simulink model "RGB_Color_Component_ManualThresholding"  (R2016a)
settings: Solver=VariableStepAuto  StartTime=0.0  StopTime=inf  RelTol=1e-3
undefined symbols (not defined in the file): none, Rec, SDTV, videoinput
libraries: visionconversions x2, imaqlib x1, visionsinks x1
settings Model: Creator=YASARA  LastModifiedBy=YASARA

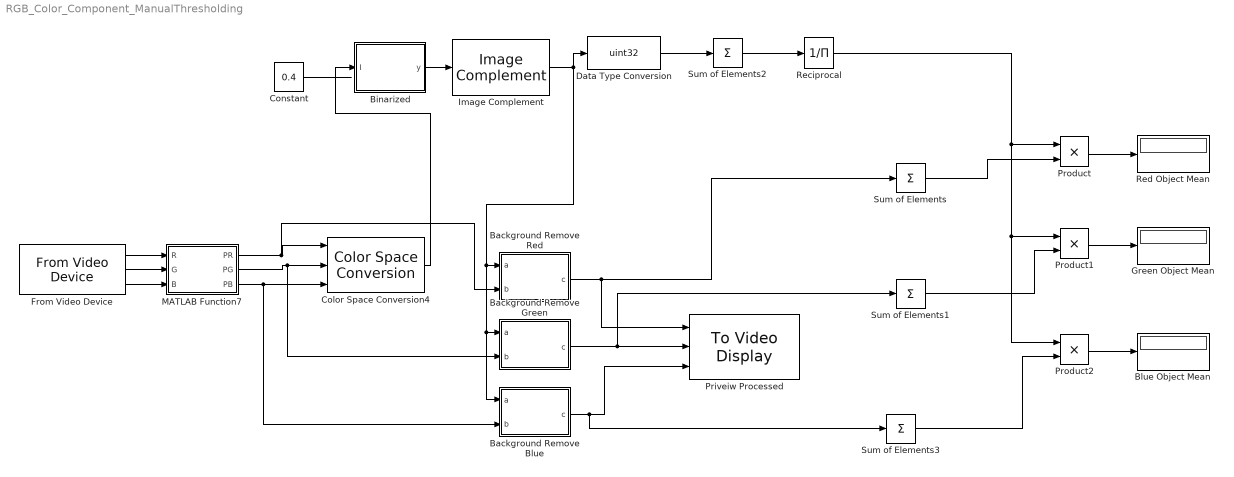
== system RGB_Color_Component_ManualThresholding ==
  Background Remove Blue : MATLAB Function  TreatAsAtomicUnit=on
  Background Remove Green : MATLAB Function  TreatAsAtomicUnit=on
  Background Remove Red : MATLAB Function  TreatAsAtomicUnit=on
  Binarized : MATLAB Function  TreatAsAtomicUnit=on
  Blue Object Mean : Display
  Color Space Conversion4 : visionconversions/Color Space  Conversion  conversion=Obsolete  conversionActive=R'G'B' to intensity  wp_str=D65  rec=Rec. 601 (SDTV)  sys=1125/60/2:1  imagePorts=Separate color signals
  Constant : Constant  Value=0.4  SampleTime=1
  Data Type Conversion : DataTypeConversion  OutDataTypeStr=uint32
  From Video Device : imaqlib/From Video Device  DeviceMenu=winvideo 1 (Integrated Webcam)  Device=winvideo 2 (USB Video Device)  ObjConstructor=videoinput('winvideo', 2)  VideoFormatMenu=YUY2_160x120  VideoFormat=YUY2_160x120  VideoSource=input1  ROIPosition=[0 0 120 160]  EnableHWTrigger=off  TriggerConfiguration=none/none  SampleTime=1/30  OutputPortsMode=Separate color signals  DataType=uint8  CanDoHWTrigger=no  ReturnedColorSpace=rgb  BlockHandle=44.0042  ROIWidth=160  ROIHeight=120  ROIColumn=0  ROIRow=0  EngXMLPath=C:\Program Files\MATLAB\R2016a\toolbox\imaq\imaq\private  DevXMLPath=C:\MATLAB\SupportPackages\R2016a\toolbox\imaq\supportpackages\genericvideo\adaptor\win64  EngLibPath=C:\Program Files\MATLAB\R2016a\toolbox\imaq\imaqblks\imaqmex\win64  ColorSpace=rgb  BayerSensorAlignment=grbg
  Green Object Mean : Display
  Image Complement : visionconversions/Image Complement
  MATLAB Function7 : MATLAB Function  TreatAsAtomicUnit=on
  Priveiw Processed : visionsinks/To Video Display  windowSizeMode=Normal  openAtMdlStart=on  fullScreen=off  videoWindowX=147  videoWindowY=157  saveWindowSize=off  videoWindowWidth=512  videoWindowHeight=384  inputColorFormat=RGB  inputType=Obsolete  imagePorts=Separate color signals  OutputDevice=On-screen video monitor  dataOrg=Column-major  isWindowOpen=off
  Product : Product
  Product1 : Product
  Product2 : Product
  Reciprocal : Product  Inputs=/  OutDataTypeStr=double  RndMeth=Simplest  SaturateOnIntegerOverflow=on
  Red Object Mean : Display
  Sum of Elements{,1..3} (4 alike) : Sum  Inputs=+  AccumDataTypeStr=uint32  OutDataTypeStr=uint32  RndMeth=Nearest
  wires:
  Binarized/1(y) -> Image Complement/1
  Color Space Conversion4/1 -> Binarized/1(I)
  Sum of Elements/1 -> Product/2
  Background Remove Red/1(c) -> Priveiw Processed/1, Sum of Elements/1
  Background Remove Green/1(c) -> Priveiw Processed/2, Sum of Elements1/1
  Background Remove Blue/1(c) -> Priveiw Processed/3, Sum of Elements3/1
  Constant/1 -> ?
  Product/1 -> Red Object Mean/1
  Sum of Elements1/1 -> Product1/2
  Product1/1 -> Green Object Mean/1
  Product2/1 -> Blue Object Mean/1
  Image Complement/1 -> Background Remove Blue/1(a), Background Remove Green/1(a), Background Remove Red/1(a), Data Type Conversion/1
  MATLAB Function7/1(PR) -> Background Remove Red/2(b), Color Space Conversion4/1
  MATLAB Function7/2(PG) -> Background Remove Green/2(b), Color Space Conversion4/2
  MATLAB Function7/3(PB) -> Background Remove Blue/2(b), Color Space Conversion4/3
  Data Type Conversion/1 -> Sum of Elements2/1
  Sum of Elements3/1 -> Product2/2
  Reciprocal/1 -> Product/1, Product1/1, Product2/1
  Sum of Elements2/1 -> Reciprocal/1
  From Video Device/1 -> MATLAB Function7/1(R)
  From Video Device/2 -> MATLAB Function7/2(G)
  From Video Device/3 -> MATLAB Function7/3(B)

== matlab function RGB_Color_Component_ManualThresholding/MATLAB Function7 ==
  data: R input; G input; PR output; B input; PG output; PB output
function [PR,PG,PB] = fcn(R,G,B)
%#codegen
Im=cat(3,R,G,B);
PR= im2double(R);
PG= im2double(G);
PB= im2double(B);
return

== matlab function RGB_Color_Component_ManualThresholding/Background Remove Green ==
  data: a input; b input; c output
function c = fcn(a,b)
%#codegen
c=uint32(a.*b);
return

== matlab function RGB_Color_Component_ManualThresholding/Binarized ==
  data: I input; y output
function y = fcn(I)
%#codegen
y=logical(I);
coder.extrinsic('graythresh');
level = graythresh(I);
BW = im2bw(I,level);

== matlab function RGB_Color_Component_ManualThresholding/Background Remove Blue ==
  data: a input; b input; c output
function c = fcn(a,b)
%#codegen
c=uint32(a.*b);
return

== matlab function RGB_Color_Component_ManualThresholding/Background Remove Red ==
  data: a input; b input; c output
function c = fcn(a,b)
%#codegen
c=uint32(a.*b);
return
